simulink model "aircraft_feedback_control_R2015a_prob_2"  (R2015b)
settings: Solver=ode45  StartTime=0.0  StopTime=10000  RelTol=1e-3
values from neighbouring files (symbols this model uses):
  aileron_step_time = 0    [RunSimLab7.m]    (also in RunSimLab7[Conflict].m)
  aileron_step_value = 0    [RunSimLab7.m]    (also in RunSimLab7[Conflict].m)
  control_surfaces_trim = control_surfaces0    [RunSimLab7.m]    (also in RunSimLab7[Conflict].m)
  DRAW_FLAG = 0    [RunSimLab7.m]    (also in RunSimLab7[Conflict].m)
  gamma_com = 1*pi/180    (= 0.0174532925199)    [RunSimLab7.m]    (also in RunSimLab7[Conflict].m = 0.0349065850399)
  gamma_trim = 0    [RunSimLab7.m]    (also in RunSimLab7[Conflict].m)
  kdg = 1    [RunSimLab7.m]    (also in RunSimLab7[Conflict].m = [.4])
  kdu = [0]    [RunSimLab7.m]    (also in RunSimLab7[Conflict].m)
  kig = 1    [RunSimLab7.m]    (also in RunSimLab7[Conflict].m = [.2])
  kiu = [0]    [RunSimLab7.m]    (also in RunSimLab7[Conflict].m = [.5])
  kpg = 1    [RunSimLab7.m]    (also in RunSimLab7[Conflict].m = [1])
  kpu = [0]    [RunSimLab7.m]    (also in RunSimLab7[Conflict].m = [.3])
  rudder_step_time = 0    [RunSimLab7.m]    (also in RunSimLab7[Conflict].m)
  rudder_step_value = 0    [RunSimLab7.m]    (also in RunSimLab7[Conflict].m)
  u_com = 1    [RunSimLab7.m]    (also in RunSimLab7[Conflict].m)
  V_trim = 21    [RunSimLab7.m]    (also in RunSimLab7[Conflict].m)
  wind_inertial = [0;0;0]    [RunSimLab7.m]    (also in RunSimLab7[Conflict].m; S_AeroForcesAndMoments.m = u(17:19,1))
undefined symbols (not defined in the file or in its folder): aircraft_parameters, FormatForFG, PlotStateVariables, S_AeroForcesAndMoments
libraries: aerolibobsolete x1, aerolibfltsims x1, aerolibatmos2 x1
settings Model: Creator=beard  LastModifiedBy=Jeremy
settings DataIOCC: SaveFormat=Array  SignalLoggingSaveFormat=ModelDataLogs
settings OptimizationCC: ExpressionDepthLimit=2147483647  InitFltsAndDblsToZero=on
settings DebuggingCC: UnderspecifiedInitializationDetection=Classic  MergeDetectMultiDrivingBlocksExec=none  SolverPrmCheckMsg=warning  FcnCallInpInsideContextMsg=UseLocalSettings  StateNameClashWarn=warning
settings HardwareCC: ProdBitPerPointer=32  ProdLargestAtomicFloat=None  ProdIntDivRoundTo=Undefined  ProdEndianess=Unspecified  ProdWordSize=32  ProdHWDeviceType=32-bit Generic
settings GRTTargetCC: GeneratePreprocessorConditionals=Disable all  CombineOutputUpdateFcns=off  GRTInterface=on
settings ConfigComp: CovModelRefEnable=Off  CovSFcnEnable=off

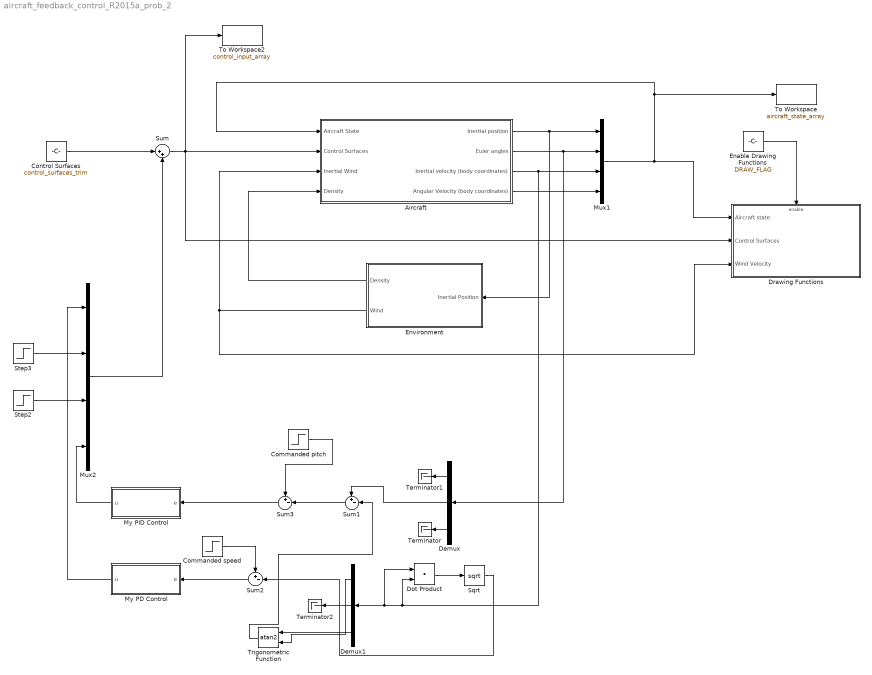
== system aircraft_feedback_control_R2015a_prob_2 ==
  Aircraft : Subsystem
  Commanded pitch : Step  Time=0  After=gamma_trim+gamma_com  SampleTime=0
  Commanded speed : Step  Time=0  After=V_trim+u_com  SampleTime=0
  Control Surfaces : Constant  Value=control_surfaces_trim
  Demux : Demux  Outputs=3
  Demux1 : Demux  Outputs=3
  Dot Product : DotProduct  InputSameDT=on  OutDataTypeStr=Inherit: Inherit via internal rule
  Drawing Functions : Subsystem  TreatAsAtomicUnit=on
  Enable Drawing Functions : Constant  Value=DRAW_FLAG
  Environment : Subsystem
  Mux1 : Mux
  Mux2 : Mux
  My PD Control : Subsystem  TreatAsAtomicUnit=on
  My PID Control : Subsystem  TreatAsAtomicUnit=on
  Sqrt : Sqrt  SaturateOnIntegerOverflow=on
  Step2 : Step  Time=rudder_step_time  After=rudder_step_value  SampleTime=0
  Step3 : Step  Time=aileron_step_time  After=aileron_step_value  SampleTime=0
  Sum : Sum  Inputs=|++
  Sum1 : Sum  Inputs=+-|
  Sum2 : Sum  Inputs=+-|
  Sum3 : Sum  Inputs=+-|
  Terminator : Terminator
  Terminator1 : Terminator
  Terminator2 : Terminator
  To Workspace : ToWorkspace  VariableName=aircraft_state_array  SaveFormat=Timeseries  SampleTime=-1
  To Workspace2 : ToWorkspace  VariableName=control_input_array  SaveFormat=Timeseries  SampleTime=-1
  Trigonometric Function : Trigonometry  Operator=atan2
  wires:
  Mux1/1 -> Drawing Functions/1(Aircraft state), Aircraft/1(Aircraft State), To Workspace/1
  Environment/1(Density) -> Aircraft/4(Density)
  Environment/2(Wind) -> Drawing Functions/3(Wind Velocity), Aircraft/3(Inertial Wind)
  Aircraft/4(Angular Velocity (body coordinates)) -> Mux1/4
  Aircraft/3(Inertial velocity (body coordinates)) -> Dot Product/2, Dot Product/1, Demux1/1, Mux1/3
  Aircraft/1(Inertial position) -> Mux1/1, Environment/1(Inertial Position)
  Enable Drawing Functions/1 -> Drawing Functions/Enable
  Mux2/1 -> Sum/2
  Step3/1 -> Mux2/2
  Step2/1 -> Mux2/3
  Control Surfaces/1 -> Sum/1
  Sum/1 -> To Workspace2/1, Drawing Functions/2(Control Surfaces), Aircraft/2(Control Surfaces)
  Aircraft/2(Euler angles) -> Demux/1, Mux1/2
  Demux/1 -> Terminator1/1
  Demux/3 -> Terminator/1
  Sum2/1 -> My PD Control/1(e)
  Commanded speed/1 -> Sum2/1
  Demux1/2 -> Terminator2/1
  Demux1/3 -> Trigonometric Function/1
  Dot Product/1 -> Sqrt/1
  Sqrt/1 -> Sum2/2
  Demux1/1 -> Trigonometric Function/2
  My PID Control/1(u) -> Mux2/4
  My PD Control/1(u) -> Mux2/1
  Demux/2 -> Sum1/1
  Trigonometric Function/1 -> Sum1/2
  Commanded pitch/1 -> Sum3/1
  Sum1/1 -> Sum3/2
  Sum3/1 -> My PID Control/1(e)

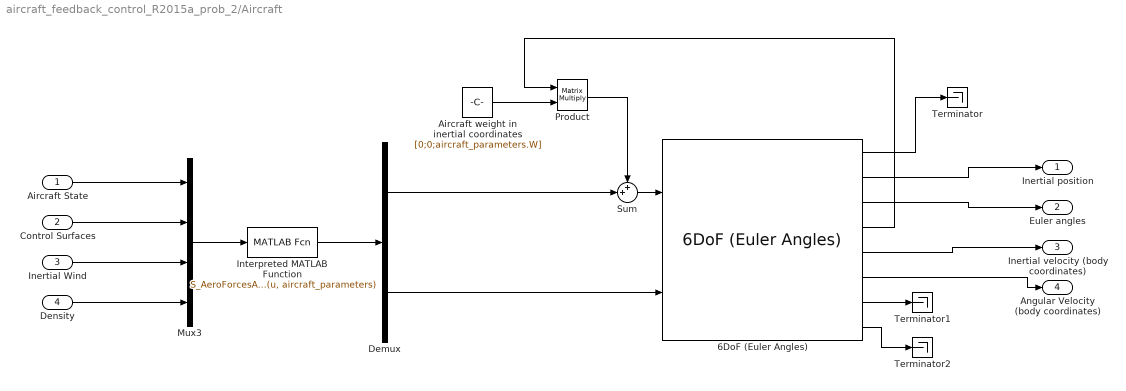
== system aircraft_feedback_control_R2015a_prob_2/Aircraft ==
  Aircraft State : Inport
  Control Surfaces : Inport  Port=2
  Inertial Wind : Inport  Port=3
  Density : Inport  Port=4
  6DoF (Euler Angles) : aerolibobsolete/6DoF (Euler Angles)  units=Metric (MKS)  mtype=Fixed  rep=Euler Angles  xme_0=position_inertial  Vm_0=velocity_body  eul_0=euler_angles  pm_0=omega_body  mass_0=aircraft_parameters.m  mass_e=0.5  mass_f=2.0  inertia=inertia_matrix  inertia_e=eye(3)  inertia_f=2*eye(3)  k_quat=1.0
  Aircraft weight in inertial coordinates : Constant  Value=[0;0;aircraft_parameters.W]
  Demux : Demux  Outputs=2
  Interpreted MATLAB Function : MATLABFcn  MATLABFcn=S_AeroForcesAndMoments(u, aircraft_parameters)  OutputDimensions=6
  Mux3 : Mux
  Product : Product  Multiplication=Matrix(*)  RndMeth=Zero
  Sum : Sum  Inputs=++|
  Terminator : Terminator
  Terminator1 : Terminator
  Terminator2 : Terminator
  Inertial position : Outport
  Euler angles : Outport  Port=2
  Inertial velocity (body coordinates) : Outport  Port=3
  Angular Velocity (body coordinates) : Outport  Port=4
  wires:
  6DoF (Euler Angles)/2 -> Inertial position/1
  6DoF (Euler Angles)/3 -> Euler angles/1
  6DoF (Euler Angles)/5 -> Inertial velocity (body coordinates)/1
  6DoF (Euler Angles)/6 -> Angular Velocity (body coordinates)/1
  6DoF (Euler Angles)/4 -> Product/1
  Sum/1 -> 6DoF (Euler Angles)/1
  Product/1 -> Sum/1
  Aircraft weight in inertial coordinates/1 -> Product/2
  Mux3/1 -> Interpreted MATLAB Function/1
  Demux/1 -> Sum/2
  Demux/2 -> 6DoF (Euler Angles)/2
  Interpreted MATLAB Function/1 -> Demux/1
  Control Surfaces/1 -> Mux3/2
  6DoF (Euler Angles)/1 -> Terminator/1
  6DoF (Euler Angles)/7 -> Terminator1/1
  6DoF (Euler Angles)/8 -> Terminator2/1
  Aircraft State/1 -> Mux3/1
  Inertial Wind/1 -> Mux3/3
  Density/1 -> Mux3/4

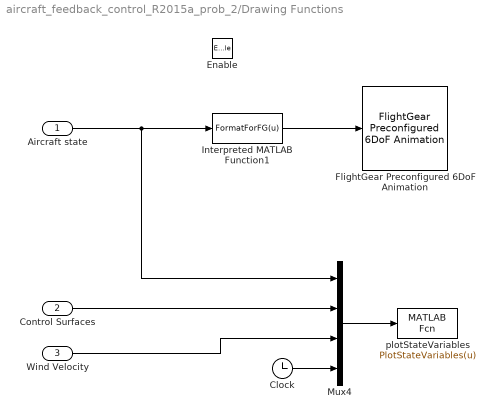
== system aircraft_feedback_control_R2015a_prob_2/Drawing Functions ==
  Aircraft state : Inport
  Control Surfaces : Inport  Port=2
  Wind Velocity : Inport  Port=3
  Enable : EnablePort
  Clock : Clock
  FlightGear Preconfigured 6DoF Animation : aerolibfltsims/FlightGear Preconfigured 6DoF Animation  xFlightGearVersion=v2.12  DestinationIpAddress=127.0.0.1  DestinationPort=5502  SampleTime=1/30
  Interpreted MATLAB Function1 : MATLABFcn  MATLABFcn=FormatForFG(u)  OutputDimensions=6
  Mux4 : Mux
  plotStateVariables : MATLABFcn  MATLABFcn=PlotStateVariables(u)  OutputDimensions=0  SampleTime=.1
  wires:
  Mux4/1 -> plotStateVariables/1
  Control Surfaces/1 -> Mux4/2
  Wind Velocity/1 -> Mux4/3
  Clock/1 -> Mux4/4
  Aircraft state/1 -> Interpreted MATLAB Function1/1, Mux4/1
  Interpreted MATLAB Function1/1 -> FlightGear Preconfigured 6DoF Animation/1

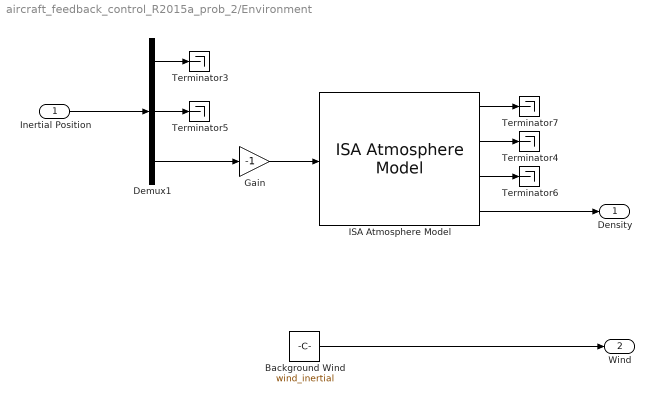
== system aircraft_feedback_control_R2015a_prob_2/Environment ==
  Inertial Position : Inport
  Background Wind : Constant  Value=wind_inertial
  Demux1 : Demux  Outputs=3
  Gain : Gain  Gain=-1
  ISA Atmosphere Model : aerolibatmos2/ISA Atmosphere Model  custom=off  g=9.80665  gamma=1.4  R=287.0531  L=0.0065  h_trop=11000  h_strat=20000  rho0=1.225  P0=101325  T0=288.15  h0=0
  Terminator{3..7} (5 alike) : Terminator
  Density : Outport
  Wind : Outport  Port=2
  wires:
  Inertial Position/1 -> Demux1/1
  Demux1/3 -> Gain/1
  Gain/1 -> ISA Atmosphere Model/1
  Demux1/1 -> Terminator3/1
  Demux1/2 -> Terminator5/1
  ISA Atmosphere Model/3 -> Terminator6/1
  ISA Atmosphere Model/2 -> Terminator4/1
  ISA Atmosphere Model/1 -> Terminator7/1
  ISA Atmosphere Model/4 -> Density/1
  Background Wind/1 -> Wind/1

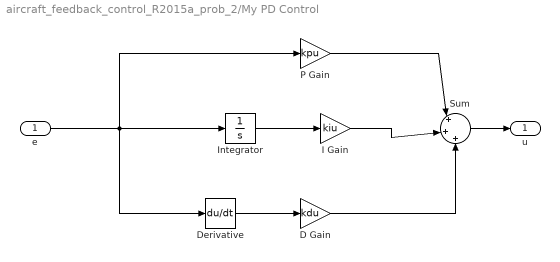
== system aircraft_feedback_control_R2015a_prob_2/My PD Control ==
  e : Inport
  D Gain : Gain  Gain=kdu
  Derivative : Derivative
  I Gain : Gain  Gain=kiu
  Integrator : Integrator
  P Gain : Gain  Gain=kpu
  Sum : Sum  Inputs=|+|+|+
  u : Outport
  wires:
  e/1 -> Integrator/1, P Gain/1, Derivative/1
  Sum/1 -> u/1
  Derivative/1 -> D Gain/1
  P Gain/1 -> Sum/1
  Integrator/1 -> I Gain/1
  D Gain/1 -> Sum/3
  I Gain/1 -> Sum/2

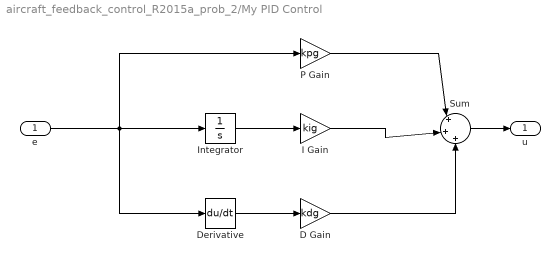
== system aircraft_feedback_control_R2015a_prob_2/My PID Control ==
  e : Inport
  D Gain : Gain  Gain=kdg
  Derivative : Derivative
  I Gain : Gain  Gain=kig
  Integrator : Integrator
  P Gain : Gain  Gain=kpg
  Sum : Sum  Inputs=|+|+|+
  u : Outport
  wires:
  e/1 -> P Gain/1, Derivative/1, Integrator/1
  Integrator/1 -> I Gain/1
  I Gain/1 -> Sum/2
  Sum/1 -> u/1
  Derivative/1 -> D Gain/1
  D Gain/1 -> Sum/3
  P Gain/1 -> Sum/1
